simulink model "WDS_with_AttackDetection"  (R2021a)
settings: Solver=FixedStepDiscrete  StartTime=0.0  StopTime=T_final  FixedStep=T_sample  RelTol=1e-3
values from neighbouring files (symbols this model uses):
  A_bar_d = readmatrix('A_bar_d.csv')    [Run_model_with_attackDetection.m]
  attack_tank_full = zeros(size(attack_tank,1),n_meas)    [Run_results.m]    (also in Run_results_new.m; time_domain_sim.m)
  b1_1 = readmatrix(append(datapath,'MLP1\b1.csv'))    [Run_model_with_attackDetection.m]
  b1_2 = readmatrix(append(datapath,'MLP2\b1.csv'))    [Run_model_with_attackDetection.m]
  b2_1 = readmatrix(append(datapath,'MLP1\b2.csv'))    [Run_model_with_attackDetection.m]
  b2_2 = readmatrix(append(datapath,'MLP2\b2.csv'))    [Run_model_with_attackDetection.m]
  b3_1 = readmatrix(append(datapath,'MLP1\b3.csv'))    [Run_model_with_attackDetection.m]
  b3_2 = readmatrix(append(datapath,'MLP2\b3.csv'))    [Run_model_with_attackDetection.m]
  b4_1 = readmatrix(append(datapath,'MLP1\b4.csv'))    [Run_model_with_attackDetection.m]
  b4_2 = readmatrix(append(datapath,'MLP2\b4.csv'))    [Run_model_with_attackDetection.m]
  B_bar_d = readmatrix('B_bar_d.csv')    [Run_model_with_attackDetection.m]
  C_obsv_d = readmatrix('C_obsv_d.csv')    [Run_model_with_attackDetection.m]
  Cm = ones(1,n_states)    [Run_model_with_attackDetection.m]
  D_obsv_d = readmatrix('D_obsv_d.csv')    [Run_model_with_attackDetection.m]
  E0_full = zeros(T,n_meas)    [Run_results.m]    (also in Run_results_new.m; time_domain_sim.m)
  eta = 0.7    [Run_model_with_attackDetection.m]
  H0_perp_full = eye(size(H0_full,1)) - H0_full*H0_full_pinv    [Run_model_with_attackDetection.m]
  I_attack_local = I_attack(1:n_attack)    [Run_results.m]    (also in Run_results_new.m; time_domain_sim.m)
  K = place(A_bar_d,B_bar_d,Pc)    [Run_model_with_attackDetection.m]
  k0 = 42    [Run_model_with_attackDetection.m]
  Lu = F-A_bar_d.'*H0_full_pinv*H1_full    [Run_model_with_attackDetection.m]
  Ly = A_bar_d.'*H0_full_pinv    [Run_model_with_attackDetection.m]
  M1 = readmatrix('M1.csv')    [Run_model_with_attackDetection.m]
  M2 = readmatrix('M2.csv')    [Run_model_with_attackDetection.m]
  n_meas = size(C_obsv_d,1)    [Run_model_with_attackDetection.m]
  offset = -inv(B_bar_d)*(A_bar_d-eye(n_states))*xd    [Run_model_with_attackDetection.m]
  p_MLP1 = load('P1.mat').P1    [Run_model_with_attackDetection.m]
  p_MLP2 = load('P2.mat').P2    [Run_model_with_attackDetection.m]
  Q0 = ones(n_meas,T)    [Run_model_with_attackDetection.m]
  T = 8    [Run_model_with_attackDetection.m]    (also in align_attack_dataset.m)
  T_sample = 0.01    [Run_model_with_attackDetection.m]
  T_start_attack = 0.1*T_final    (= 0.8)    [Run_model_with_attackDetection.m]
  T_start_detect = T_start_attack+T*T_sample    (= 0.88)    [Run_model_with_attackDetection.m]
  tau2 = readmatrix('tau2.csv')    [Run_model_with_attackDetection.m]
  U0 = zeros(n_int,T+1)    [Run_model_with_attackDetection.m]
  w1_1 = readmatrix(append(datapath,'\MLP1\w1.csv'))    [Run_model_with_attackDetection.m]
  w1_2 = readmatrix(append(datapath,'\MLP2\w1.csv'))    [Run_model_with_attackDetection.m]
  w2_1 = readmatrix(append(datapath,'MLP1\w2.csv'))    [Run_model_with_attackDetection.m]
  w2_2 = readmatrix(append(datapath,'MLP2\w2.csv'))    [Run_model_with_attackDetection.m]
  w3_1 = readmatrix(append(datapath,'MLP1\w3.csv'))    [Run_model_with_attackDetection.m]
  w3_2 = readmatrix(append(datapath,'MLP2\w3.csv'))    [Run_model_with_attackDetection.m]
  w4_1 = readmatrix(append(datapath,'MLP1\w4.csv'))    [Run_model_with_attackDetection.m]
  w4_2 = readmatrix(append(datapath,'MLP2\w4.csv'))    [Run_model_with_attackDetection.m]
  x0 = 0.3+ 0.2*rand(n_states,1)    [Run_model_with_attackDetection.m]
  xd = 0.5*ones(n_states,1)    [Run_model_with_attackDetection.m]
  Y0 = zeros(n_meas,T)    [Run_model_with_attackDetection.m]
undefined symbols (not defined in the file or in its folder): F, H0_full, H1_full, n_int, n_states, T_start_opt
libraries: simulink x15
(part 1 of 2)
settings Model: Creator=zysgh  LastModifiedBy=Abelb

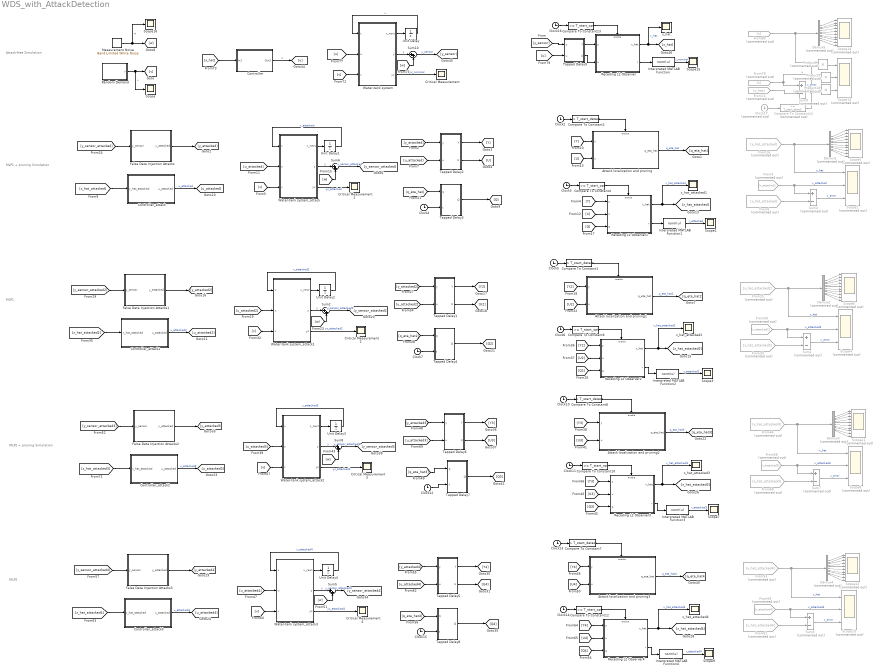
== system WDS_with_AttackDetection ==
  note: MLP1 + pruning Simulation
  note: MLP1
  note: MLP2 + pruning Simulation
  note: MLP2
  note: Attack-free Simulation
  Attack localization and pruning : Subsystem
  Attack localization and pruning1 : Subsystem
  Attack localization and pruning2 : Subsystem
  Attack localization and pruning3 : Subsystem
  Clock{2..7,10..16} (13 alike) : Clock
  Clock17 : Clock  Commented=on
  Compare To Constant{1..2,7..8} (4 alike) : simulink/Logic and Bit Operations/Compare To Constant  relop=>  const=T_start_detect  OutDataTypeStr=boolean
  Compare To Constant{4,6,10,12..13} (5 alike) : simulink/Logic and Bit Operations/Compare To Constant  relop=>=  const=T_start_opt  OutDataTypeStr=boolean
  Compare To Constant14 : simulink/Logic and Bit Operations/Compare To Constant  Commented=on  relop=>=  const=T_start_attack  OutDataTypeStr=boolean
  Controller : Subsystem
  Controller_attack : Subsystem
  Controller_attack1 : Subsystem
  Controller_attack2 : Subsystem
  Controller_attack3 : Subsystem
  Critical Measurement{,1..4} (5 alike) : Scope
  Demux{1..5} (5 alike) : Demux  Commented=on  Outputs=n_states
  False Data Injection Attacks : Subsystem
  False Data Injection Attacks1 : Subsystem
  False Data Injection Attacks2 : Subsystem
  False Data Injection Attacks3 : Subsystem
  From16 : From  Commented=on  GotoTag=x_hat_attacked
  From25 : From  Commented=on  GotoTag=x_hat_attacked2
  From3 : From  Commented=on  GotoTag=x_attacked
  From30 : From  Commented=on  GotoTag=x_attacked2
  From33 : From  Commented=on  GotoTag=x_hat_attacked2
  From44 : From  Commented=on  GotoTag=x_hat_attacked3
  From53 : From  Commented=on  GotoTag=x_hat_attacked4
  From58 : From  Commented=on  GotoTag=x_attacked3
  From59 : From  Commented=on  GotoTag=x_attacked4
  From6 : From  Commented=on  GotoTag=x_hat_attacked
  From61 : From  Commented=on  GotoTag=x_hat_attacked4
  From68 : From  Commented=on  GotoTag=x_hat_attacked3
  From74 : From  Commented=on  GotoTag=x_hat
  From78 : From  Commented=on  GotoTag=x
  From80 : From  Commented=on  GotoTag=x
  Interpreted MATLAB Function{,1..4} (5 alike) : MATLABFcn  MATLABFcn=norm(u)
  Measurement Noise : simulink/Sources/Band-Limited White Noise  Cov=[0.001]  Ts=T_sample  seed=[23341]
  Product10 : Product  Commented=on
  Product8 : Product  Commented=on
  Product9 : Product  Commented=on
  Random Demand : Subsystem
  Receding L2 Observer : Subsystem
  Receding L2 Observer1 : Subsystem
  Receding L2 Observer2 : Subsystem
  Receding L2 Observer3 : Subsystem
  Receding L2 Observer4 : Subsystem
  Scope{,1,3,7,9,15..16} (7 alike) : Scope
  Scope{2,4,8,10,13} (5 alike) : Scope  Commented=on  NumInputPorts=3
  Scope{5..6,11..12,14} (5 alike) : Scope  Commented=on  NumInputPorts=10
  Sum{1,3..4,7,9} (5 alike) : Sum  Commented=on  Inputs=+-
  Sum{2,5..6,8,10} (5 alike) : Sum  Inputs=|++
  Tapped Delay1 : Subsystem
  Tapped Delay2 : Subsystem
  Tapped Delay3 : Subsystem
  Tapped Delay4 : Subsystem
  Tapped Delay5 : Subsystem
  Tapped Delay6 : Subsystem
  Tapped Delay7 : Subsystem
  Tapped Delay8 : Subsystem
  Tapped Delay9 : Subsystem
  Unit Delay{,1..4} (5 alike) : UnitDelay  InitialCondition=x0  SampleTime=-1  HasFrameUpgradeWarning=on
  Water-tank system : MATLAB Function  TreatAsAtomicUnit=on
  Water-tank system_attack : MATLAB Function  TreatAsAtomicUnit=on
  Water-tank system_attack1 : MATLAB Function  TreatAsAtomicUnit=on
  Water-tank system_attack2 : MATLAB Function  TreatAsAtomicUnit=on
  Water-tank system_attack3 : MATLAB Function  TreatAsAtomicUnit=on
  x_hat : Scope
  x_hat_attacked{1..4} (4 alike) : Scope
  wires:
  Demux1/10 -> Scope5/10
  Tapped Delay3/1(Q) -> [Q]
  Water-tank system_attack/1(x_next) -> Unit Delay1/1
  [x_hat_attacked] -> Controller_attack/1(x_hat_attacked)
  Clock2/1 -> Compare To Constant2/1
  Unit Delay1/1 -> Water-tank system_attack/1(x)  "x_attacked"
  Water-tank system_attack/2(y) -> Sum6/1  "y"
  Controller_attack/1(u_attacked) -> [u_attacked]  "u_attacked"
  Clock4/1 -> Tapped Delay3/2(t)
  Tapped Delay2/1(Y) -> [Y]
  [v] -> Water-tank system_attack/3(v)
  [w] -> Sum6/2
  [y_attacked] -> Tapped Delay2/1(y)
  [U] -> Attack localization and pruning/2(u)
  [Y] -> Attack localization and pruning/1(y)
  [u_attacked] -> Water-tank system_attack/2(u)
  False Data Injection Attacks/1(y_attacked) -> [y_attacked]
  Tapped Delay2/2(U) -> [U]
  Random Demand/1(v) -> Scope/1, [v]  "v"
  Compare To Constant2/1 -> Attack localization and pruning/Enable
  [q_eta_hat] -> Tapped Delay3/1(q)
  [u_attacked] -> Tapped Delay2/2(u)
  Demux1/4 -> Scope5/4
  Sum6/1 -> [y_sensor_attacked]  "y_sensor_attacked"
  Attack localization and pruning/1(q_eta_hat) -> [q_eta_hat]  "q_eta_hat"
  Measurement Noise/1 -> Scope16/1, [w]  "w"
  Demux1/2 -> Scope5/2
  From3/1 -> Sum4/1, Scope2/2  "x_attacked"
  From16/1 -> Demux1/1, Scope2/1  "x_hat"
  Demux1/6 -> Scope5/6
  Demux1/9 -> Scope5/9
  Demux1/7 -> Scope5/7
  [y_sensor_attacked] -> False Data Injection Attacks/1(y_sensor)
  Demux1/1 -> Scope5/1
  Demux1/8 -> Scope5/8
  Demux1/5 -> Scope5/5
  Demux1/3 -> Scope5/3
  Sum4/1 -> Scope2/3  "x_error"
  From6/1 -> Sum4/2
  Interpreted MATLAB Function1/1 -> Scope1/1  "r_attacked"
  Compare To Constant4/1 -> Receding L2 Observer1/Enable
  Receding L2 Observer1/1(x_hat) -> x_hat_attacked1/1, [x_hat_attacked]  "x_hat_attacked"
  Receding L2 Observer1/2(r) -> Interpreted MATLAB Function1/1
  Clock3/1 -> Compare To Constant4/1
  [Y] -> Receding L2 Observer1/1(y)
  [Q] -> Receding L2 Observer1/3(q)
  [U] -> Receding L2 Observer1/2(u)
  Demux2/1 -> Scope6/1
  Demux2/9 -> Scope6/9
  [U2] -> Receding L2 Observer2/2(u)
  [q_eta_hat2] -> Tapped Delay4/1(q)
  Demux2/3 -> Scope6/3
  Receding L2 Observer2/1(x_hat) -> x_hat_attacked2/1, [x_hat_attacked2]  "x_hat_attacked2"
  [y_sensor_attacked2] -> False Data Injection Attacks1/1(y_sensor)
  Demux2/8 -> Scope6/8
  Clock6/1 -> Compare To Constant6/1
  [Q2] -> Receding L2 Observer2/3(q)
  Controller_attack1/1(u_attacked) -> [u_attacked2]  "u_attacked2"
  [y_attacked2] -> Tapped Delay1/1(y)
  Sum1/1 -> Scope4/3  "x_error"
  Interpreted MATLAB Function2/1 -> Scope3/1  "r_attacked2"
  Demux2/5 -> Scope6/5
  Demux2/7 -> Scope6/7
  [u_attacked2] -> Water-tank system_attack1/2(u)
  From33/1 -> Sum1/2
  Sum2/1 -> [y_sensor_attacked2]  "y_sensor_attacked2"
  Demux2/2 -> Scope6/2
  [w] -> Sum2/2
  From30/1 -> Sum1/1, Scope4/2  "x_attacked2"
  From25/1 -> Demux2/1, Scope4/1  "x_hat"
  [v] -> Water-tank system_attack1/3(v)
  Compare To Constant6/1 -> Receding L2 Observer2/Enable
  [u_attacked2] -> Tapped Delay1/2(u)
  Attack localization and pruning1/1(q_eta_hat) -> [q_eta_hat2]  "q_eta_hat2"
  False Data Injection Attacks1/1(y_attacked) -> [y_attacked2]
  Unit Delay2/1 -> Water-tank system_attack1/1(x)  "x_attacked2"
  Tapped Delay1/2(U) -> [U2]
  [U2] -> Attack localization and pruning1/2(u)
  Compare To Constant1/1 -> Attack localization and pruning1/Enable
  [Y2] -> Attack localization and pruning1/1(y)
  Demux2/4 -> Scope6/4
  Receding L2 Observer2/2(r) -> Interpreted MATLAB Function2/1
  Clock5/1 -> Compare To Constant1/1
  [Y2] -> Receding L2 Observer2/1(y)
  Tapped Delay4/1(Q) -> [Q2]
  Clock7/1 -> Tapped Delay4/2(t)
  Water-tank system_attack1/1(x_next) -> Unit Delay2/1
  Tapped Delay1/1(Y) -> [Y2]
  Water-tank system_attack1/2(y) -> Sum2/1  "y"
  Demux2/10 -> Scope6/10
  Demux2/6 -> Scope6/6
  [x_hat_attacked2] -> Controller_attack1/1(x_hat_attacked)
  Demux3/1 -> Scope11/1
  Demux3/9 -> Scope11/9
  [U3] -> Receding L2 Observer3/2(u)
  Tapped Delay6/2(U) -> [U3]
  [q_eta_hat3] -> Tapped Delay7/1(q)
  Demux3/3 -> Scope11/3
  [Q3] -> Receding L2 Observer3/3(q)
  Sum8/1 -> [y_sensor_attacked3]  "y_sensor_attacked3"
  Receding L2 Observer3/1(x_hat) -> x_hat_attacked3/1, [x_hat_attacked3]  "x_hat_attacked3"
  [y_sensor_attacked3] -> False Data Injection Attacks2/1(y_sensor)
  [w] -> Sum8/2
  Demux3/5 -> Scope11/5
  Compare To Constant10/1 -> Receding L2 Observer3/Enable
  From68/1 -> Sum7/2
  Demux3/8 -> Scope11/8
  [Y3] -> Receding L2 Observer3/1(y)
  Clock11/1 -> Compare To Constant10/1
  Controller_attack2/1(u_attacked) -> [u_attacked3]  "u_attacked3"
  [v] -> Water-tank system_attack2/3(v)
  [y_attacked3] -> Tapped Delay6/1(y)
  Attack localization and pruning2/1(q_eta_hat) -> [q_eta_hat3]  "q_eta_hat3"
  Sum7/1 -> Scope8/3  "x_error"
  Interpreted MATLAB Function3/1 -> Scope7/1  "r_attacked3"
  Demux3/7 -> Scope11/7
  From58/1 -> Sum7/1, Scope8/2  "x_attacked3"
  Receding L2 Observer3/2(r) -> Interpreted MATLAB Function3/1
  Demux3/6 -> Scope11/6
  Demux3/2 -> Scope11/2
  From44/1 -> Demux3/1, Scope8/1  "x_hat"
  False Data Injection Attacks2/1(y_attacked) -> [y_attacked3]
  Unit Delay3/1 -> Water-tank system_attack2/1(x)  "x_attacked3"
  [U3] -> Attack localization and pruning2/2(u)
  [Y3] -> Attack localization and pruning2/1(y)
  Demux3/4 -> Scope11/4
  Clock10/1 -> Compare To Constant8/1
  Tapped Delay7/1(Q) -> [Q3]
  Tapped Delay6/1(Y) -> [Y3]
  Clock12/1 -> Tapped Delay7/2(t)
  [x_hat_attacked3] -> Controller_attack2/1(x_hat_attacked)
  Water-tank system_attack2/1(x_next) -> Unit Delay3/1
  Water-tank system_attack2/2(y) -> Sum8/1  "y"
  Demux3/10 -> Scope11/10
  Controller_attack3/1(u_attacked) -> [u_attacked4]  "u_attacked4"
  [y_attacked4] -> Tapped Delay5/1(y)
  Sum3/1 -> Scope10/3  "x_error"
  Demux4/8 -> Scope12/8
  Clock14/1 -> Compare To Constant12/1
  Demux4/3 -> Scope12/3
  Demux4/9 -> Scope12/9
  [Y4] -> Receding L2 Observer4/1(y)
  Tapped Delay5/1(Y) -> [Y4]
  Water-tank system_attack3/1(x_next) -> Unit Delay4/1
  Clock15/1 -> Tapped Delay8/2(t)
  Clock13/1 -> Compare To Constant7/1
  Receding L2 Observer4/2(r) -> Interpreted MATLAB Function4/1
  Tapped Delay8/1(Q) -> [Q4]
  Compare To Constant7/1 -> Attack localization and pruning3/Enable
  Demux4/4 -> Scope12/4
  [Y4] -> Attack localization and pruning3/1(y)
  [U4] -> Attack localization and pruning3/2(u)
  Tapped Delay5/2(U) -> [U4]
  [u_attacked4] -> Tapped Delay5/2(u)
  [u_attacked3] -> Water-tank system_attack2/2(u)
  Compare To Constant12/1 -> Receding L2 Observer4/Enable
  [q_eta_hat4] -> Tapped Delay8/1(q)
  False Data Injection Attacks3/1(y_attacked) -> [y_attacked4]
  From53/1 -> Demux4/1, Scope10/1  "x_hat"
  [Q4] -> Receding L2 Observer4/3(q)
  Demux4/1 -> Scope12/1
  From59/1 -> Sum3/1, Scope10/2  "x_attacked4"
  [v] -> Water-tank system_attack3/3(v)
  Unit Delay4/1 -> Water-tank system_attack3/1(x)  "x_attacked4"
  Demux4/2 -> Scope12/2
  [w] -> Sum5/2
  Compare To Constant8/1 -> Attack localization and pruning2/Enable
  Interpreted MATLAB Function4/1 -> Scope9/1  "r_attacked4"
  Demux4/7 -> Scope12/7
  Receding L2 Observer4/1(x_hat) -> x_hat_attacked4/1, [x_hat_attacked4]  "x_hat_attacked4"
  From61/1 -> Sum3/2
  Sum5/1 -> [y_sensor_attacked4]  "y_sensor_attacked4"
  [u_attacked4] -> Water-tank system_attack3/2(u)
  Demux4/5 -> Scope12/5
  [y_sensor_attacked4] -> False Data Injection Attacks3/1(y_sensor)
  [x_hat_attacked4] -> Controller_attack3/1(x_hat_attacked)
  Demux4/10 -> Scope12/10
  [u_attacked3] -> Tapped Delay6/2(u)
  Water-tank system_attack3/2(y) -> Sum5/1  "y"
  [U4] -> Receding L2 Observer4/2(u)
  Demux4/6 -> Scope12/6
  Attack localization and pruning3/1(q_eta_hat) -> [q_eta_hat4]  "q_eta_hat4"
  Demux5/7 -> Scope14/7
  Water-tank system/2(y) -> Sum10/1  "y"
  Demux5/1 -> Scope14/1
  [u] -> Tapped Delay9/2(u)
  [v] -> Water-tank system/3(v)
  Demux5/5 -> Scope14/5
  From80/1 -> Product8/1, Demux5/1
  Product8/1 -> Scope13/1
  From78/1 -> Product9/1, Sum9/1  "x"
  Demux5/10 -> Scope14/10
  From74/1 -> Sum9/2
  Product10/1 -> Scope13/3
  Sum9/1 -> Product10/1  "x_error"
  Demux5/2 -> Scope14/2
  Demux5/8 -> Scope14/8
  Tapped Delay9/2(U) -> Receding L2 Observer/2(u)
  Unit Delay/1 -> Water-tank system/1(x)  "x"
  Water-tank system/1(x_next) -> Unit Delay/1
  Clock17/1 -> Compare To Constant14/1
  Product9/1 -> Scope13/2
  Controller/1(Out1) -> [u]  "u"
  Sum10/1 -> [y_sensor]  "y_sensor"
  Demux5/6 -> Scope14/6
  [x_hat] -> Controller/1(In1)
  [w] -> Sum10/2
  [u] -> Water-tank system/2(u)
  Interpreted MATLAB Function/1 -> Scope15/1  "r_nominal"
  Demux5/3 -> Scope14/3
  Receding L2 Observer/2(r) -> Interpreted MATLAB Function/1
  Compare To Constant14/1 -> Product10/2, Product9/2, Product8/2
  Receding L2 Observer/1(x_hat) -> x_hat/1, [x_hat]  "x_hat"
  Demux5/9 -> Scope14/9
  Demux5/4 -> Scope14/4
  Tapped Delay9/1(Y) -> Receding L2 Observer/1(y)
  Compare To Constant13/1 -> Receding L2 Observer/Enable
  Clock16/1 -> Compare To Constant13/1
  Water-tank system/3(yc) -> Critical Measurement/1  "yc_nominal"
  Water-tank system_attack1/3(yc) -> Critical Measurement2/1  "yc_attacked2"
  Water-tank system_attack2/3(yc) -> Critical Measurement3/1  "yc_attacked3"
  Water-tank system_attack3/3(yc) -> Critical Measurement4/1  "yc_attacked4"
  Water-tank system_attack/3(yc) -> Critical Measurement1/1  "yc_attacked"
  [y_sensor] -> Tapped Delay9/1(y)

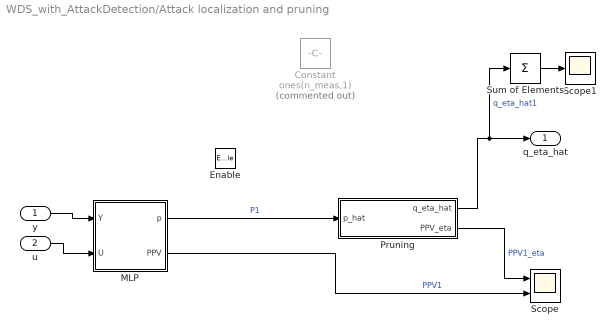
== system WDS_with_AttackDetection/Attack localization and pruning ==
  y : Inport
  u : Inport  Port=2
  Enable : EnablePort
  Constant : Constant  Commented=on  Value=ones(n_meas,1)
  MLP : MATLAB Function  TreatAsAtomicUnit=on
  Pruning : MATLAB Function  TreatAsAtomicUnit=on
  Scope : Scope  NumInputPorts=2
  Scope1 : Scope
  Sum of Elements : Sum  Inputs=+
  q_eta_hat : Outport
  wires:
  y/1 -> MLP/1(Y)
  u/1 -> MLP/2(U)
  Pruning/1(q_eta_hat) -> Sum of Elements/1, q_eta_hat/1  "q_eta_hat1"
  MLP/2(PPV) -> Scope/2  "PPV1"
  Pruning/2(PPV_eta) -> Scope/1  "PPV1_eta"
  MLP/1(p) -> Pruning/1(p_hat)  "P1"
  Sum of Elements/1 -> Scope1/1

== system WDS_with_AttackDetection/Attack localization and pruning1 ==
  y : Inport
  u : Inport  Port=2
  Enable : EnablePort
  MLP : MATLAB Function  TreatAsAtomicUnit=on
  Scope : Scope
  Sum of Elements : Sum  Inputs=+
  q_eta_hat : Outport
  wires:
  y/1 -> MLP/1(Y)
  u/1 -> MLP/2(U)
  MLP/1(q_hat) -> q_eta_hat/1, Sum of Elements/1
  Sum of Elements/1 -> Scope/1

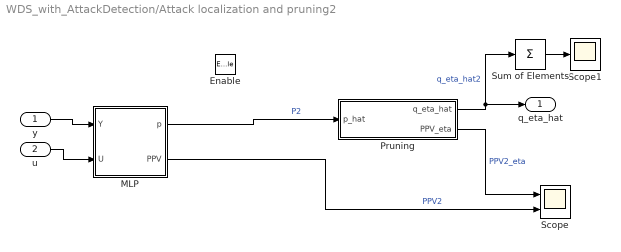
== system WDS_with_AttackDetection/Attack localization and pruning2 ==
  y : Inport
  u : Inport  Port=2
  Enable : EnablePort
  MLP : MATLAB Function  TreatAsAtomicUnit=on
  Pruning : MATLAB Function  TreatAsAtomicUnit=on
  Scope : Scope  NumInputPorts=2
  Scope1 : Scope
  Sum of Elements : Sum  Inputs=+
  q_eta_hat : Outport
  wires:
  y/1 -> MLP/1(Y)
  u/1 -> MLP/2(U)
  MLP/2(PPV) -> Scope/2  "PPV2"
  Pruning/2(PPV_eta) -> Scope/1  "PPV2_eta"
  MLP/1(p) -> Pruning/1(p_hat)  "P2"
  Pruning/1(q_eta_hat) -> Sum of Elements/1, q_eta_hat/1  "q_eta_hat2"
  Sum of Elements/1 -> Scope1/1

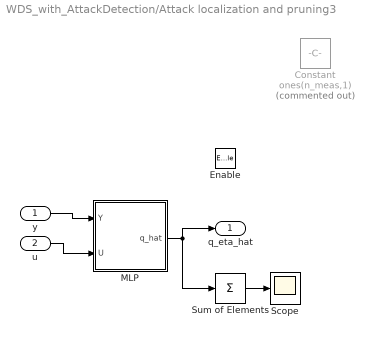
== system WDS_with_AttackDetection/Attack localization and pruning3 ==
  y : Inport
  u : Inport  Port=2
  Enable : EnablePort
  Constant : Constant  Commented=on  Value=ones(n_meas,1)
  MLP : MATLAB Function  TreatAsAtomicUnit=on
  Scope : Scope
  Sum of Elements : Sum  Inputs=+
  q_eta_hat : Outport
  wires:
  y/1 -> MLP/1(Y)
  u/1 -> MLP/2(U)
  MLP/1(q_hat) -> q_eta_hat/1, Sum of Elements/1
  Sum of Elements/1 -> Scope/1

== system WDS_with_AttackDetection/Controller ==
  In1 : Inport
  Constant : Constant  Value=offset
  Constant1 : Constant  Value=xd
  Gain : Gain  Gain=-K  Multiplication=Matrix(K*u) (u vector)
  Scope : Scope
  Sum : Sum  Inputs=|+-
  Sum3 : Sum  Inputs=|++
  Out1 : Outport
  wires:
  Sum3/1 -> Out1/1, Scope/1  "u"
  Constant/1 -> Sum3/2
  Constant1/1 -> Sum/2
  Gain/1 -> Sum3/1  "u"
  Sum/1 -> Gain/1
  In1/1 -> Sum/1

== system WDS_with_AttackDetection/Controller_attack ==
  x_hat_attacked : Inport
  Constant2 : Constant  Value=offset
  Constant3 : Constant  Value=xd
  Gain1 : Gain  Gain=-K  Multiplication=Matrix(K*u) (u vector)
  Scope7 : Scope
  Sum7 : Sum  Inputs=|+-
  Sum8 : Sum  Inputs=|++
  u_attacked : Outport
  wires:
  x_hat_attacked/1 -> Sum7/1
  Sum7/1 -> Gain1/1
  Gain1/1 -> Sum8/1
  Constant2/1 -> Sum8/2
  Sum8/1 -> u_attacked/1, Scope7/1  "u_attacked"
  Constant3/1 -> Sum7/2

== system WDS_with_AttackDetection/Controller_attack1 ==
  x_hat_attacked : Inport
  Constant2 : Constant  Value=offset
  Constant3 : Constant  Value=xd
  Gain1 : Gain  Gain=-K  Multiplication=Matrix(K*u) (u vector)
  Scope7 : Scope
  Sum7 : Sum  Inputs=|+-
  Sum8 : Sum  Inputs=|++
  u_attacked : Outport
  wires:
  x_hat_attacked/1 -> Sum7/1
  Sum7/1 -> Gain1/1
  Gain1/1 -> Sum8/1
  Constant2/1 -> Sum8/2
  Sum8/1 -> u_attacked/1, Scope7/1  "u_attacked"
  Constant3/1 -> Sum7/2

== system WDS_with_AttackDetection/Controller_attack2 ==
  x_hat_attacked : Inport
  Constant2 : Constant  Value=offset
  Constant3 : Constant  Value=xd
  Gain1 : Gain  Gain=-K  Multiplication=Matrix(K*u) (u vector)
  Scope7 : Scope
  Sum7 : Sum  Inputs=|+-
  Sum8 : Sum  Inputs=|++
  u_attacked : Outport
  wires:
  x_hat_attacked/1 -> Sum7/1
  Sum7/1 -> Gain1/1
  Gain1/1 -> Sum8/1
  Constant2/1 -> Sum8/2
  Sum8/1 -> u_attacked/1, Scope7/1  "u_attacked"
  Constant3/1 -> Sum7/2

== system WDS_with_AttackDetection/Controller_attack3 ==
  x_hat_attacked : Inport
  Constant2 : Constant  Value=offset
  Constant3 : Constant  Value=xd
  Gain1 : Gain  Gain=-K  Multiplication=Matrix(K*u) (u vector)
  Scope7 : Scope
  Sum7 : Sum  Inputs=|+-
  Sum8 : Sum  Inputs=|++
  u_attacked : Outport
  wires:
  x_hat_attacked/1 -> Sum7/1
  Sum7/1 -> Gain1/1
  Gain1/1 -> Sum8/1
  Constant2/1 -> Sum8/2
  Sum8/1 -> u_attacked/1, Scope7/1  "u_attacked"
  Constant3/1 -> Sum7/2

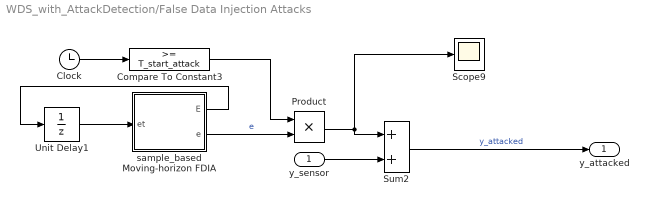
== system WDS_with_AttackDetection/False Data Injection Attacks ==
  y_sensor : Inport
  Clock : Clock
  Compare To Constant3 : simulink/Logic and Bit Operations/Compare To Constant  relop=>=  const=T_start_attack  OutDataTypeStr=boolean
  Product : Product
  Scope9 : Scope
  Sum2 : Sum
  Unit Delay1 : UnitDelay  InitialCondition=E0_full.'  SampleTime=-1  HasFrameUpgradeWarning=on
  sample_based Moving-horizon FDIA : MATLAB Function  TreatAsAtomicUnit=on
  y_attacked : Outport
  wires:
  Compare To Constant3/1 -> Product/1
  y_sensor/1 -> Sum2/2
  Product/1 -> Sum2/1, Scope9/1
  Clock/1 -> Compare To Constant3/1
  Sum2/1 -> y_attacked/1  "y_attacked"
  sample_based Moving-horizon FDIA/1(E) -> Unit Delay1/1
  sample_based Moving-horizon FDIA/2(e) -> Product/2  "e"
  Unit Delay1/1 -> sample_based Moving-horizon FDIA/1(et)

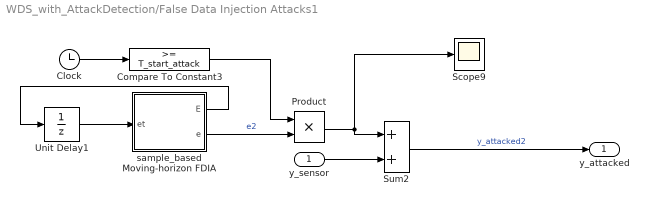
== system WDS_with_AttackDetection/False Data Injection Attacks1 ==
  y_sensor : Inport
  Clock : Clock
  Compare To Constant3 : simulink/Logic and Bit Operations/Compare To Constant  relop=>=  const=T_start_attack  OutDataTypeStr=boolean
  Product : Product
  Scope9 : Scope
  Sum2 : Sum
  Unit Delay1 : UnitDelay  InitialCondition=E0_full.'  SampleTime=-1  HasFrameUpgradeWarning=on
  sample_based Moving-horizon FDIA : MATLAB Function  TreatAsAtomicUnit=on
  y_attacked : Outport
  wires:
  sample_based Moving-horizon FDIA/2(e) -> Product/2  "e2"
  Unit Delay1/1 -> sample_based Moving-horizon FDIA/1(et)
  Product/1 -> Sum2/1, Scope9/1
  y_sensor/1 -> Sum2/2
  Compare To Constant3/1 -> Product/1
  Sum2/1 -> y_attacked/1  "y_attacked2"
  Clock/1 -> Compare To Constant3/1
  sample_based Moving-horizon FDIA/1(E) -> Unit Delay1/1

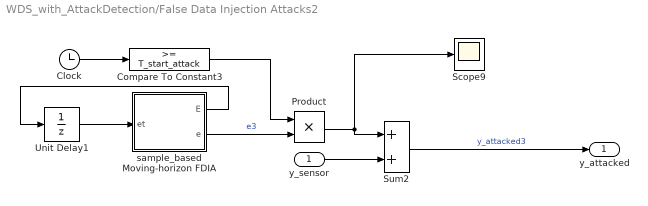
== system WDS_with_AttackDetection/False Data Injection Attacks2 ==
  y_sensor : Inport
  Clock : Clock
  Compare To Constant3 : simulink/Logic and Bit Operations/Compare To Constant  relop=>=  const=T_start_attack  OutDataTypeStr=boolean
  Product : Product
  Scope9 : Scope
  Sum2 : Sum
  Unit Delay1 : UnitDelay  InitialCondition=E0_full.'  SampleTime=-1  HasFrameUpgradeWarning=on
  sample_based Moving-horizon FDIA : MATLAB Function  TreatAsAtomicUnit=on
  y_attacked : Outport
  wires:
  Sum2/1 -> y_attacked/1  "y_attacked3"
  sample_based Moving-horizon FDIA/1(E) -> Unit Delay1/1
  Clock/1 -> Compare To Constant3/1
  Compare To Constant3/1 -> Product/1
  Product/1 -> Sum2/1, Scope9/1
  Unit Delay1/1 -> sample_based Moving-horizon FDIA/1(et)
  y_sensor/1 -> Sum2/2
  sample_based Moving-horizon FDIA/2(e) -> Product/2  "e3"

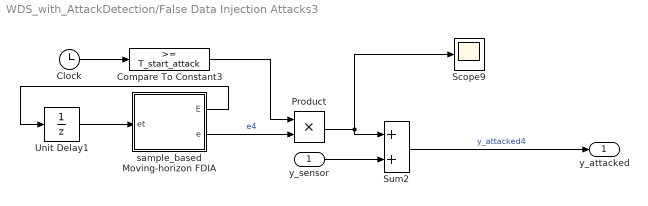
== system WDS_with_AttackDetection/False Data Injection Attacks3 ==
  y_sensor : Inport
  Clock : Clock
  Compare To Constant3 : simulink/Logic and Bit Operations/Compare To Constant  relop=>=  const=T_start_attack  OutDataTypeStr=boolean
  Product : Product
  Scope9 : Scope
  Sum2 : Sum
  Unit Delay1 : UnitDelay  InitialCondition=E0_full.'  SampleTime=-1  HasFrameUpgradeWarning=on
  sample_based Moving-horizon FDIA : MATLAB Function  TreatAsAtomicUnit=on
  y_attacked : Outport
  wires:
  Sum2/1 -> y_attacked/1  "y_attacked4"
  sample_based Moving-horizon FDIA/1(E) -> Unit Delay1/1
  Clock/1 -> Compare To Constant3/1
  Compare To Constant3/1 -> Product/1
  Product/1 -> Sum2/1, Scope9/1
  Unit Delay1/1 -> sample_based Moving-horizon FDIA/1(et)
  y_sensor/1 -> Sum2/2
  sample_based Moving-horizon FDIA/2(e) -> Product/2  "e4"

== system WDS_with_AttackDetection/Random Demand ==
  " random demand" : MATLAB Function  TreatAsAtomicUnit=on
  Product4 : Product
  Pulse Generator : DiscretePulseGenerator  Period=10  SampleTime=T_sample
  v : Outport
  wires:
  " random demand"/1(v) -> Product4/2
  Product4/1 -> v/1
  Pulse Generator/1 -> Product4/1

== system WDS_with_AttackDetection/Receding L2 Observer ==
  y : Inport
  u : Inport  Port=2
  Enable : EnablePort
  ResilientOptimzer : MATLAB Function  TreatAsAtomicUnit=on
  x_hat : Outport
  r : Outport  Port=2
  wires:
  u/1 -> [U]
  y/1 -> ResilientOptimzer/2(Y)
  [U] -> ResilientOptimzer/1(U)
  ResilientOptimzer/1(x_next) -> x_hat/1
  ResilientOptimzer/2(r) -> r/1

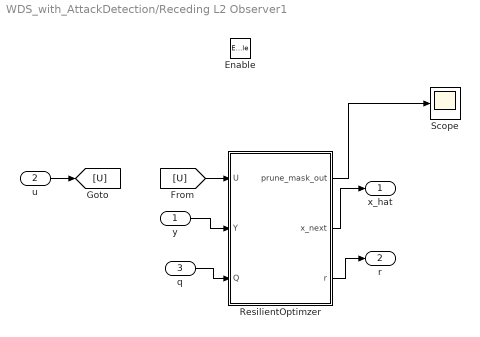
== system WDS_with_AttackDetection/Receding L2 Observer1 ==
  y : Inport
  u : Inport  Port=2
  q : Inport  Port=3
  Enable : EnablePort
  ResilientOptimzer : MATLAB Function  TreatAsAtomicUnit=on
  Scope : Scope
  x_hat : Outport
  r : Outport  Port=2
  wires:
  u/1 -> [U]
  y/1 -> ResilientOptimzer/2(Y)
  [U] -> ResilientOptimzer/1(U)
  ResilientOptimzer/2(x_next) -> x_hat/1
  ResilientOptimzer/3(r) -> r/1
  ResilientOptimzer/1(prune_mask_out) -> Scope/1
  q/1 -> ResilientOptimzer/3(Q)

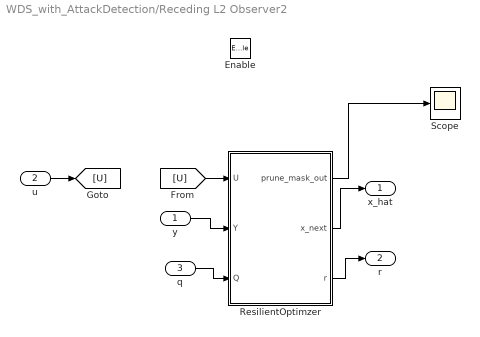
== system WDS_with_AttackDetection/Receding L2 Observer2 ==
  y : Inport
  u : Inport  Port=2
  q : Inport  Port=3
  Enable : EnablePort
  ResilientOptimzer : MATLAB Function  TreatAsAtomicUnit=on
  Scope : Scope
  x_hat : Outport
  r : Outport  Port=2
  wires:
  u/1 -> [U]
  y/1 -> ResilientOptimzer/2(Y)
  [U] -> ResilientOptimzer/1(U)
  ResilientOptimzer/2(x_next) -> x_hat/1
  ResilientOptimzer/3(r) -> r/1
  ResilientOptimzer/1(prune_mask_out) -> Scope/1
  q/1 -> ResilientOptimzer/3(Q)

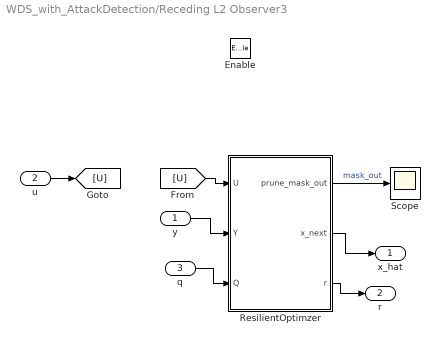
== system WDS_with_AttackDetection/Receding L2 Observer3 ==
  y : Inport
  u : Inport  Port=2
  q : Inport  Port=3
  Enable : EnablePort
  ResilientOptimzer : MATLAB Function  TreatAsAtomicUnit=on
  Scope : Scope
  x_hat : Outport
  r : Outport  Port=2
  wires:
  u/1 -> [U]
  y/1 -> ResilientOptimzer/2(Y)
  [U] -> ResilientOptimzer/1(U)
  ResilientOptimzer/2(x_next) -> x_hat/1
  ResilientOptimzer/3(r) -> r/1
  ResilientOptimzer/1(prune_mask_out) -> Scope/1  "mask_out"
  q/1 -> ResilientOptimzer/3(Q)

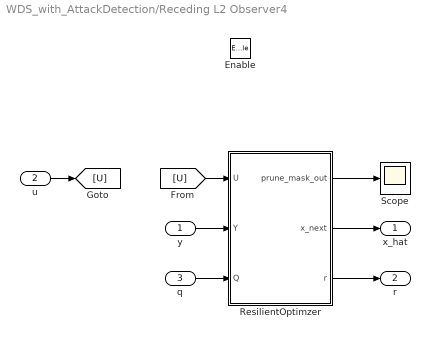
== system WDS_with_AttackDetection/Receding L2 Observer4 ==
  y : Inport
  u : Inport  Port=2
  q : Inport  Port=3
  Enable : EnablePort
  ResilientOptimzer : MATLAB Function  TreatAsAtomicUnit=on
  Scope : Scope
  x_hat : Outport
  r : Outport  Port=2
  wires:
  u/1 -> [U]
  y/1 -> ResilientOptimzer/2(Y)
  [U] -> ResilientOptimzer/1(U)
  ResilientOptimzer/2(x_next) -> x_hat/1
  ResilientOptimzer/3(r) -> r/1
  ResilientOptimzer/1(prune_mask_out) -> Scope/1
  q/1 -> ResilientOptimzer/3(Q)

== system WDS_with_AttackDetection/Tapped Delay1 ==
  y : Inport
  u : Inport  Port=2
  Unit Delay : UnitDelay  InitialCondition=U0  SampleTime=-1  HasFrameUpgradeWarning=on
  Unit Delay1 : UnitDelay  InitialCondition=Y0  SampleTime=-1  HasFrameUpgradeWarning=on
  tapped_delay : MATLAB Function  TreatAsAtomicUnit=on
  Y : Outport
  U : Outport  Port=2
  wires:
  u/1 -> tapped_delay/1(u)
  y/1 -> tapped_delay/3(y)
  tapped_delay/1(U) -> Unit Delay/1, U/1
  tapped_delay/2(Y) -> Unit Delay1/1, Y/1
  Unit Delay/1 -> tapped_delay/2(ut)
  Unit Delay1/1 -> tapped_delay/4(yt)

== system WDS_with_AttackDetection/Tapped Delay2 ==
  y : Inport
  u : Inport  Port=2
  Unit Delay : UnitDelay  InitialCondition=U0  SampleTime=-1  HasFrameUpgradeWarning=on
  Unit Delay1 : UnitDelay  InitialCondition=Y0  SampleTime=-1  HasFrameUpgradeWarning=on
  tapped_delay : MATLAB Function  TreatAsAtomicUnit=on
  Y : Outport
  U : Outport  Port=2
  wires:
  u/1 -> tapped_delay/1(u)
  y/1 -> tapped_delay/3(y)
  tapped_delay/1(U) -> Unit Delay/1, U/1
  tapped_delay/2(Y) -> Unit Delay1/1, Y/1
  Unit Delay/1 -> tapped_delay/2(ut)
  Unit Delay1/1 -> tapped_delay/4(yt)

== system WDS_with_AttackDetection/Tapped Delay3 ==
  q : Inport
  t : Inport  Port=2
  Unit Delay1 : UnitDelay  InitialCondition=Q0  SampleTime=-1  HasFrameUpgradeWarning=on
  tapped_delay1 : MATLAB Function  TreatAsAtomicUnit=on
  Q : Outport
  wires:
  t/1 -> tapped_delay1/1(t)
  Unit Delay1/1 -> tapped_delay1/3(qt)
  tapped_delay1/1(Q) -> Q/1, Unit Delay1/1
  q/1 -> tapped_delay1/2(q)

== system WDS_with_AttackDetection/Tapped Delay4 ==
  q : Inport
  t : Inport  Port=2
  Unit Delay1 : UnitDelay  InitialCondition=Q0  SampleTime=-1  HasFrameUpgradeWarning=on
  tapped_delay1 : MATLAB Function  TreatAsAtomicUnit=on
  Q : Outport
  wires:
  t/1 -> tapped_delay1/1(t)
  Unit Delay1/1 -> tapped_delay1/3(qt)
  tapped_delay1/1(Q) -> Q/1, Unit Delay1/1
  q/1 -> tapped_delay1/2(q)

== system WDS_with_AttackDetection/Tapped Delay5 ==
  y : Inport
  u : Inport  Port=2
  Unit Delay : UnitDelay  InitialCondition=U0  SampleTime=-1  HasFrameUpgradeWarning=on
  Unit Delay1 : UnitDelay  InitialCondition=Y0  SampleTime=-1  HasFrameUpgradeWarning=on
  tapped_delay : MATLAB Function  TreatAsAtomicUnit=on
  Y : Outport
  U : Outport  Port=2
  wires:
  u/1 -> tapped_delay/1(u)
  y/1 -> tapped_delay/3(y)
  tapped_delay/1(U) -> Unit Delay/1, U/1
  tapped_delay/2(Y) -> Unit Delay1/1, Y/1
  Unit Delay/1 -> tapped_delay/2(ut)
  Unit Delay1/1 -> tapped_delay/4(yt)

== system WDS_with_AttackDetection/Tapped Delay6 ==
  y : Inport
  u : Inport  Port=2
  Unit Delay : UnitDelay  InitialCondition=U0  SampleTime=-1  HasFrameUpgradeWarning=on
  Unit Delay1 : UnitDelay  InitialCondition=Y0  SampleTime=-1  HasFrameUpgradeWarning=on
  tapped_delay : MATLAB Function  TreatAsAtomicUnit=on
  Y : Outport
  U : Outport  Port=2
  wires:
  u/1 -> tapped_delay/1(u)
  y/1 -> tapped_delay/3(y)
  tapped_delay/1(U) -> Unit Delay/1, U/1
  tapped_delay/2(Y) -> Unit Delay1/1, Y/1
  Unit Delay/1 -> tapped_delay/2(ut)
  Unit Delay1/1 -> tapped_delay/4(yt)

== system WDS_with_AttackDetection/Tapped Delay7 ==
  q : Inport
  t : Inport  Port=2
  Unit Delay1 : UnitDelay  InitialCondition=Q0  SampleTime=-1  HasFrameUpgradeWarning=on
  tapped_delay1 : MATLAB Function  TreatAsAtomicUnit=on
  Q : Outport
  wires:
  Unit Delay1/1 -> tapped_delay1/3(qt)
  t/1 -> tapped_delay1/1(t)
  tapped_delay1/1(Q) -> Q/1, Unit Delay1/1
  q/1 -> tapped_delay1/2(q)

== system WDS_with_AttackDetection/Tapped Delay8 ==
  q : Inport
  t : Inport  Port=2
  Unit Delay1 : UnitDelay  InitialCondition=Q0  SampleTime=-1  HasFrameUpgradeWarning=on
  tapped_delay1 : MATLAB Function  TreatAsAtomicUnit=on
  Q : Outport
  wires:
  t/1 -> tapped_delay1/1(t)
  Unit Delay1/1 -> tapped_delay1/3(qt)
  tapped_delay1/1(Q) -> Q/1, Unit Delay1/1  "Q"
  q/1 -> tapped_delay1/2(q)

== system WDS_with_AttackDetection/Tapped Delay9 ==
  y : Inport
  u : Inport  Port=2
  Unit Delay : UnitDelay  InitialCondition=U0  SampleTime=-1  HasFrameUpgradeWarning=on
  Unit Delay1 : UnitDelay  InitialCondition=Y0  SampleTime=-1  HasFrameUpgradeWarning=on
  tapped_delay : MATLAB Function  TreatAsAtomicUnit=on
  Y : Outport
  U : Outport  Port=2
  wires:
  u/1 -> tapped_delay/1(u)
  y/1 -> tapped_delay/3(y)
  tapped_delay/1(U) -> Unit Delay/1, U/1
  tapped_delay/2(Y) -> Unit Delay1/1, Y/1
  Unit Delay/1 -> tapped_delay/2(ut)
  Unit Delay1/1 -> tapped_delay/4(yt)

== matlab function WDS_with_AttackDetection/Attack localization and pruning/MLP ==
  data: Y input; p output; U input; n_meas parameter; n_int parameter; T parameter; w1_1 parameter; w2_1 parameter; w3_1 parameter; b1_1 parameter; PPV output; I_attack_local parameter; b2_1 parameter; b3_1 parameter; w4_1 parameter; b4_1 parameter
function [p,PPV] = fcn(Y,U,n_meas,n_int,T,w1_1,w2_1, w3_1, b1_1,I_attack_local, b2_1, b3_1,w4_1, b4_1)

%% Unpacking data
u_local = zeros(n_int,T+1-1);
u_local(:,:) = U(:,1:end-1);
u = u_local(:);
y = Y(:);

% prepare input data for MLP
input = [y ; u];


%% prediction
% q_hat = ones(n_meas,1);
% coder.extrinsic('MLP_realtime')
% q_hat = MLP_realtime(Y,u_local,n_meas);

q_hat_prob =  execute_mlp_4layers(input,w1_1,w2_1,w3_1,w4_1,b1_1,b2_1,b3_1,b4_1);
q_hat = q_hat_prob;
q_hat(q_hat<0.5) = 0;
q_hat(q_hat>=0.5)= 1;
p = q_hat_prob;

q = ones(n_meas,1);
q(I_attack_local) = 0;
PPV = sum(q.*q_hat)/sum(q_hat);

end

== matlab function WDS_with_AttackDetection/Attack localization and pruning/Pruning ==
  data: p_hat input; q_eta_hat output; eta parameter; n_meas parameter; PPV_eta output; I_attack_local parameter; p_MLP1 parameter; k0 parameter
function [q_eta_hat,PPV_eta] = fcn(p_hat,eta, n_meas, I_attack_local, p_MLP1,k0)

q_eta_hat = ones(n_meas,1);
coder.extrinsic('pruning_algorithm2')
q_eta_hat = pruning_algorithm2(p_hat,p_MLP1,eta,k0);

q = ones(n_meas,1);
q(I_attack_local) = 0;
PPV_eta = sum(q.*q_eta_hat)/sum(q_eta_hat);
end

== matlab function WDS_with_AttackDetection/Tapped Delay3/tapped_delay1 ==
  data: t input; q input; qt input; Q output; n_meas parameter; T_start_detect parameter; T parameter
function Q  = fcn(t, q,qt,n_meas,T_start_detect, T)
%% tapped_delay_array
% shift columns from tapped matrix to the left and appends most recent
% vector to the last column
% %%% input
% ut(:,1:end-1) = ut(:,2:end);
% ut(:,end) = u;
% U = ut;
% %%% output
% yt(:,1:end-1) = yt(:,2:end);
% yt(:,end) = y;
% Y = yt;
%%% pruning support
Q = ones(n_meas,T);
if t>T_start_detect
    qt(:,1:end-1) = qt(:,2:end);
    qt(:,end) = q;
    Q = qt;
end
end

== matlab function WDS_with_AttackDetection/Receding L2 Observer/ResilientOptimzer ==
  data: x_next output; U input; Y input; Ly parameter; Lu parameter; H0_perp_full parameter; H1_full parameter; r output
function [x_next,r]  = fcn(U,Y, Ly, Lu,H0_perp_full, H1_full)


u_local = U(:,1:end-1);
% vectorized
u = u_local(:);
y = Y(:);

x_next = zeros(10,1);
x_next(:) = Ly*y + Lu*u;

r = H0_perp_full*(y-H1_full*u);

== matlab function WDS_with_AttackDetection/Receding L2 Observer2/ResilientOptimzer ==
  data: prune_mask_out output; x_next output; U input; Y input; Q input; n_int parameter; T parameter; H0_perp_full parameter; H0_full parameter; r output; n_states parameter; H1_full parameter; F parameter; A_bar_d parameter
function [prune_mask_out,x_next,r]  = fcn(U,Y,Q,n_int,T,H0_perp_full,H0_full, n_states, H1_full,F, A_bar_d)

u_local = zeros(n_int,T+1-1);
u_local(:,:) = U(:,1:end-1);
% vectorized
u = u_local(:);
y = Y(:);
q_eta_hat = Q(:);

%% pruning
prune_mask_out = sum(q_eta_hat>0.5);   % mask for safe nodes
prune_mask = find(q_eta_hat>0.5); %find(q_eta_hat>0.5); % true(size(q_eta_hat,1),1);

H0_eta = H0_full(prune_mask,:);
H1_eta = H1_full(prune_mask,:);

H0_eta_pinv = pinv(H0_eta,0.001);
Ly = A_bar_d.'*H0_eta_pinv;
Lu = F-A_bar_d.'*H0_eta_pinv*H1_eta;

x_next = zeros(n_states,1);
x_next(:) = Ly*y(prune_mask) + Lu*u;

r = H0_perp_full*(y-H1_full*u);

== matlab function WDS_with_AttackDetection/Tapped Delay1/tapped_delay ==
  data: u input; U output; ut input; y input; yt input; Y output
function [U,Y] = fcn(u,ut,y,yt)
%% tapped_delay_array
% shift columns from tapped matrix to the left and appends most recent
% vector to the last column
%%% input
ut(:,1:end-1) = ut(:,2:end);
ut(:,end) = u;
U = ut;
%%% output
yt(:,1:end-1) = yt(:,2:end);
yt(:,end) = y;
Y = yt;

== matlab function WDS_with_AttackDetection/Tapped Delay4/tapped_delay1 ==
  data: t input; q input; qt input; Q output; n_meas parameter; T_start_detect parameter; T parameter
function Q  = fcn(t, q,qt,n_meas,T_start_detect, T)
%% tapped_delay_array
% shift columns from tapped matrix to the left and appends most recent
% vector to the last column
% %%% input
% ut(:,1:end-1) = ut(:,2:end);
% ut(:,end) = u;
% U = ut;
% %%% output
% yt(:,1:end-1) = yt(:,2:end);
% yt(:,end) = y;
% Y = yt;
%%% pruning support
Q = ones(n_meas,T);
if t>T_start_detect
    qt(:,1:end-1) = qt(:,2:end);
    qt(:,end) = q;
    Q = qt;
end
end

== matlab function WDS_with_AttackDetection/Water-tank system_attack1 ==
  data: x input; x_next output; u input; v input; y output; A_bar_d parameter; C_obsv_d parameter; B_bar_d parameter; D_obsv_d parameter; yc output; Cm parameter
function [x_next,y,yc] = fcn(x,u,v,A_bar_d,C_obsv_d,B_bar_d,D_obsv_d,Cm)
% Discrete state-space model for system

x_next = A_bar_d*x + B_bar_d*u - v;

y = C_obsv_d*x + D_obsv_d*u;

% critical measurements
yc = Cm*x;

== matlab function WDS_with_AttackDetection/Attack localization and pruning2/MLP ==
  data: Y input; p output; U input; n_meas parameter; n_int parameter; T parameter; w1_2 parameter; w2_2 parameter; w3_2 parameter; b1_2 parameter; PPV output; I_attack_local parameter; b2_2 parameter; b3_2 parameter; w4_2 parameter; b4_2 parameter
function [p,PPV] = fcn(Y,U,n_meas,n_int,T,w1_2,w2_2, w3_2, b1_2,I_attack_local, b2_2, b3_2,w4_2, b4_2)

%% Unpacking data
u_local = zeros(n_int,T+1-1);
u_local(:,:) = U(:,1:end-1);
u = u_local(:);
y = Y(:);

% prepare input data for MLP
input = [y ; u];


%% prediction
% q_hat = ones(n_meas,1);
% coder.extrinsic('MLP_realtime')
% q_hat = MLP_realtime(Y,u_local,n_meas);

q_hat_prob = execute_mlp_4layers(input,w1_2,w2_2,w3_2,w4_2,b1_2,b2_2,b3_2,b4_2);
q_hat = q_hat_prob;
q_hat(q_hat<0.5) = 0;
q_hat(q_hat>=0.5)= 1;
p = q_hat_prob;

q = ones(n_meas,1);
q(I_attack_local) = 0;
PPV = sum(q.*q_hat)/sum(q_hat);

end

== matlab function WDS_with_AttackDetection/Attack localization and pruning2/Pruning ==
  data: p_hat input; q_eta_hat output; eta parameter; n_meas parameter; PPV_eta output; I_attack_local parameter; p_MLP2 parameter; k0 parameter
function [q_eta_hat,PPV_eta] = fcn(p_hat,eta, n_meas, I_attack_local, p_MLP2,k0)

q_eta_hat = ones(n_meas,1);
coder.extrinsic('pruning_algorithm2')
q_eta_hat = pruning_algorithm2(p_hat,p_MLP2,eta,k0);

q = ones(n_meas,1);
q(I_attack_local) = 0;
PPV_eta = sum(q.*q_eta_hat)/sum(q_eta_hat);
end

== matlab function WDS_with_AttackDetection/Attack localization and pruning3/MLP ==
  data: Y input; q_hat output; U input; n_int parameter; T parameter; w1_2 parameter; w2_2 parameter; w3_2 parameter; b1_2 parameter; b2_2 parameter; b3_2 parameter; w4_2 parameter; b4_2 parameter
function q_hat = fcn(Y,U,n_int,T,w1_2,w2_2, w3_2,b1_2, b2_2, b3_2,w4_2, b4_2)

%% Unpacking data
u_local = zeros(n_int,T+1-1);
u_local(:,:) = U(:,1:end-1);
u = u_local(:);
y = Y(:);

% prepare input data for MLP
input = [y ; u];


%% prediction
% q_hat = ones(n_meas,1);
% coder.extrinsic('MLP_realtime')
% q_hat = MLP_realtime(Y,u_local,n_meas);

q_hat_prob = execute_mlp_4layers(input,w1_2,w2_2,w3_2,w4_2,b1_2,b2_2,b3_2,b4_2);
q_hat = q_hat_prob;
q_hat(q_hat<0.5) = 0;
q_hat(q_hat>=0.5)= 1;

end

== matlab function WDS_with_AttackDetection/Receding L2 Observer3/ResilientOptimzer ==
  data: prune_mask_out output; x_next output; U input; Y input; Q input; n_int parameter; T parameter; H0_perp_full parameter; H0_full parameter; r output; n_states parameter; H1_full parameter; F parameter; A_bar_d parameter
function [prune_mask_out,x_next,r]  = fcn(U,Y,Q,n_int,T,H0_perp_full,H0_full, n_states, H1_full,F, A_bar_d)

u_local = zeros(n_int,T+1-1);
u_local(:,:) = U(:,1:end-1);
% vectorized
u = u_local(:);
y = Y(:);
q_eta_hat = Q(:);

%% pruning
prune_mask_out = sum(q_eta_hat>0.5);   % mask for safe nodes
prune_mask = find(q_eta_hat>0.5); %find(q_eta_hat>0.5); % true(size(q_eta_hat,1),1);

H0_eta = H0_full(prune_mask,:);
H1_eta = H1_full(prune_mask,:);

H0_eta_pinv = pinv(H0_eta,0.001);
Ly = A_bar_d.'*H0_eta_pinv;
Lu = F-A_bar_d.'*H0_eta_pinv*H1_eta;

x_next = zeros(n_states,1);
x_next(:) = Ly*y(prune_mask) + Lu*u;

r = H0_perp_full*(y-H1_full*u);

== matlab function WDS_with_AttackDetection/Receding L2 Observer4/ResilientOptimzer ==
  data: prune_mask_out output; x_next output; U input; Y input; Q input; n_int parameter; T parameter; H0_perp_full parameter; H0_full parameter; r output; n_states parameter; H1_full parameter; F parameter; A_bar_d parameter
function [prune_mask_out,x_next,r]  = fcn(U,Y,Q,n_int,T,H0_perp_full,H0_full, n_states, H1_full,F, A_bar_d)

u_local = zeros(n_int,T+1-1);
u_local(:,:) = U(:,1:end-1);
% vectorized
u = u_local(:);
y = Y(:);
q_eta_hat = Q(:);

%% pruning
prune_mask_out = sum(q_eta_hat>0.5);   % mask for safe nodes
prune_mask = find(q_eta_hat>0.5); %find(q_eta_hat>0.5); % true(size(q_eta_hat,1),1);

H0_eta = H0_full(prune_mask,:);
H1_eta = H1_full(prune_mask,:);

H0_eta_pinv = pinv(H0_eta,0.001);
Ly = A_bar_d.'*H0_eta_pinv;
Lu = F-A_bar_d.'*H0_eta_pinv*H1_eta;

x_next = zeros(n_states,1);
x_next(:) = Ly*y(prune_mask) + Lu*u;

r = H0_perp_full*(y-H1_full*u);

== matlab function WDS_with_AttackDetection/Tapped Delay5/tapped_delay ==
  data: u input; U output; ut input; y input; yt input; Y output
function [U,Y] = fcn(u,ut,y,yt)
%% tapped_delay_array
% shift columns from tapped matrix to the left and appends most recent
% vector to the last column
%%% input
ut(:,1:end-1) = ut(:,2:end);
ut(:,end) = u;
U = ut;
%%% output
yt(:,1:end-1) = yt(:,2:end);
yt(:,end) = y;
Y = yt;

== matlab function WDS_with_AttackDetection/Tapped Delay6/tapped_delay ==
  data: u input; U output; ut input; y input; yt input; Y output
function [U,Y] = fcn(u,ut,y,yt)
%% tapped_delay_array
% shift columns from tapped matrix to the left and appends most recent
% vector to the last column
%%% input
ut(:,1:end-1) = ut(:,2:end);
ut(:,end) = u;
U = ut;
%%% output
yt(:,1:end-1) = yt(:,2:end);
yt(:,end) = y;
Y = yt;

== matlab function WDS_with_AttackDetection/Tapped Delay8/tapped_delay1 ==
  data: t input; q input; qt input; Q output; n_meas parameter; T_start_detect parameter; T parameter
function Q  = fcn(t, q,qt,n_meas,T_start_detect, T)
%% tapped_delay_array
% shift columns from tapped matrix to the left and appends most recent
% vector to the last column
% %%% input
% ut(:,1:end-1) = ut(:,2:end);
% ut(:,end) = u;
% U = ut;
% %%% output
% yt(:,1:end-1) = yt(:,2:end);
% yt(:,end) = y;
% Y = yt;
%%% pruning support
Q = ones(n_meas,T);
if t>T_start_detect
    qt(:,1:end-1) = qt(:,2:end);
    qt(:,end) = q;
    Q = qt;
end
end

== matlab function WDS_with_AttackDetection/Tapped Delay9/tapped_delay ==
  data: u input; U output; ut input; y input; yt input; Y output
function [U,Y] = fcn(u,ut,y,yt)
%% tapped_delay_array
% shift columns from tapped matrix to the left and appends most recent
% vector to the last column
%%% input
ut(:,1:end-1) = ut(:,2:end);
ut(:,end) = u;
U = ut;
%%% output
yt(:,1:end-1) = yt(:,2:end);
yt(:,end) = y;
Y = yt;

== matlab function WDS_with_AttackDetection/Attack localization and pruning1/MLP ==
  data: Y input; q_hat output; U input; n_int parameter; T parameter; w1_1 parameter; w2_1 parameter; w3_1 parameter; b1_1 parameter; b2_1 parameter; b3_1 parameter; w4_1 parameter; b4_1 parameter
function q_hat = fcn(Y,U,n_int,T,w1_1,w2_1, w3_1, b1_1, b2_1, b3_1, w4_1, b4_1)

%% Unpacking data
u_local = zeros(n_int,T+1-1);
u_local(:,:) = U(:,1:end-1);
u = u_local(:);
y = Y(:);

% prepare input data for MLP
input = [y ; u];


%% prediction
% q_hat = ones(n_meas,1);
% coder.extrinsic('MLP_realtime')
% q_hat = MLP_realtime(Y,u_local,n_meas);

q_hat_prob =  execute_mlp_4layers(input,w1_1,w2_1,w3_1,w4_1,b1_1,b2_1,b3_1,b4_1);
q_hat = q_hat_prob;
q_hat(q_hat<0.5) = 0;
q_hat(q_hat>=0.5)= 1;

end

== matlab function WDS_with_AttackDetection/Water-tank system_attack2 ==
  data: x input; x_next output; u input; v input; y output; A_bar_d parameter; C_obsv_d parameter; B_bar_d parameter; D_obsv_d parameter; yc output; Cm parameter
function [x_next,y,yc] = fcn(x,u,v,A_bar_d,C_obsv_d,B_bar_d,D_obsv_d,Cm)
% Discrete state-space model for system

x_next = A_bar_d*x + B_bar_d*u - v;

y = C_obsv_d*x + D_obsv_d*u;

% critical measurements
yc = Cm*x;

== matlab function WDS_with_AttackDetection/Water-tank system_attack3 ==
  data: x input; x_next output; u input; v input; y output; A_bar_d parameter; C_obsv_d parameter; B_bar_d parameter; D_obsv_d parameter; yc output; Cm parameter
function [x_next,y,yc] = fcn(x,u,v,A_bar_d,C_obsv_d,B_bar_d,D_obsv_d,Cm)
% Discrete state-space model for system

x_next = A_bar_d*x + B_bar_d*u - v;

y = C_obsv_d*x + D_obsv_d*u;

% critical measurements
yc = Cm*x;

== matlab function WDS_with_AttackDetection/False Data Injection Attacks/sample_based Moving-horizon FDIA ==
  data: E output; e output double; et input; attack_tank_full parameter; M1 parameter; M2 parameter; tau2 parameter; T parameter
function [E,e] = fcn(et, attack_tank_full, M1, M2,tau2,T)
%% function [E,e] = fcn(et, attack_tank_full, M1, M2,tau2)
% sample-based moving horizon FDIA
% optimization problem or returns zeros if infeasible:
%         Maximize: ||M1*[e_history; e_i]||_2 
%         Subject to: ||M2*[e_history; e_i||_2 <= tau
%                      e_i \in e_data
% Inputs: 
%         - et [n_meas-by-T]         : cahce
%         - attack_tank_full [N_data-by-n_meas]: tank of pre-generated attacks
%         - M1 [n_m1-by-(T*n_meas)]  : Attack impact operator
%         - M2 [n_m2-by-(T*n_meas)]  : Detection residual operator
%         - tau2 [scalar]            : Detection threshold
% Output:
%         - E [n_meas-by-T] : cahce
%         - e [n_meas-by-1] : current-time-step attack
%
% Yu zheng, RASLab, FAMU-FSU College of Engineering, Tallahassee, 2021, Aug.



%% get T-1 attacks history
E_history = et(:,2:end).';  % [n_meas-by-(T-1)]
e_history = E_history(:);  % [n_meas*(T-1)-by-1]

%% get current attack
e = getCurrentAttack(e_history,M1,M2,tau2,attack_tank_full,T);

%% update cache E (save T recent attacks)
et(:,1:end-1) = et(:,2:end);
et(:,end) = e;
E = et;

== matlab function WDS_with_AttackDetection/False Data Injection Attacks1/sample_based Moving-horizon FDIA ==
  data: E output; e output double; et input; attack_tank_full parameter; M1 parameter; M2 parameter; tau2 parameter; T parameter
function [E,e] = fcn(et, attack_tank_full, M1, M2,tau2,T)
%% function [E,e] = fcn(et, attack_tank_full, M1, M2,tau2)
% sample-based moving horizon FDIA
% optimization problem or returns zeros if infeasible:
%         Maximize: ||M1*[e_history; e_i]||_2 
%         Subject to: ||M2*[e_history; e_i||_2 <= tau
%                      e_i \in e_data
% Inputs: 
%         - et [n_meas-by-T]         : cahce
%         - attack_tank_full [N_data-by-n_meas]: tank of pre-generated attacks
%         - M1 [n_m1-by-(T*n_meas)]  : Attack impact operator
%         - M2 [n_m2-by-(T*n_meas)]  : Detection residual operator
%         - tau2 [scalar]            : Detection threshold
% Output:
%         - E [n_meas-by-T] : cahce
%         - e [n_meas-by-1] : current-time-step attack
%
% Yu zheng, RASLab, FAMU-FSU College of Engineering, Tallahassee, 2021, Aug.



%% get T-1 attacks history
E_history = et(:,2:end).';  % [n_meas-by-(T-1)]
e_history = E_history(:);  % [n_meas*(T-1)-by-1]

%% get current attack
e = getCurrentAttack(e_history,M1,M2,tau2,attack_tank_full,T);

%% update cache E (save T recent attacks)
et(:,1:end-1) = et(:,2:end);
et(:,end) = e;
E = et;

== matlab function WDS_with_AttackDetection/False Data Injection Attacks2/sample_based Moving-horizon FDIA ==
  data: E output; e output double; et input; attack_tank_full parameter; M1 parameter; M2 parameter; tau2 parameter; T parameter
function [E,e] = fcn(et, attack_tank_full, M1, M2,tau2,T)
%% function [E,e] = fcn(et, attack_tank_full, M1, M2,tau2)
% sample-based moving horizon FDIA
% optimization problem or returns zeros if infeasible:
%         Maximize: ||M1*[e_history; e_i]||_2 
%         Subject to: ||M2*[e_history; e_i||_2 <= tau
%                      e_i \in e_data
% Inputs: 
%         - et [n_meas-by-T]         : cahce
%         - attack_tank_full [N_data-by-n_meas]: tank of pre-generated attacks
%         - M1 [n_m1-by-(T*n_meas)]  : Attack impact operator
%         - M2 [n_m2-by-(T*n_meas)]  : Detection residual operator
%         - tau2 [scalar]            : Detection threshold
% Output:
%         - E [n_meas-by-T] : cahce
%         - e [n_meas-by-1] : current-time-step attack
%
% Yu zheng, RASLab, FAMU-FSU College of Engineering, Tallahassee, 2021, Aug.



%% get T-1 attacks history
E_history = et(:,2:end).';  % [n_meas-by-(T-1)]
e_history = E_history(:);  % [n_meas*(T-1)-by-1]

%% get current attack
e = getCurrentAttack(e_history,M1,M2,tau2,attack_tank_full,T);

%% update cache E (save T recent attacks)
et(:,1:end-1) = et(:,2:end);
et(:,end) = e;
E = et;
